simulink model "AC_Voltage_Controller_Bidirectional_L_Load"  (R2021b)
settings: Solver=ode23tb  StartTime=0.0  StopTime=0.1  MaxStep=1e-4  RelTol=1e-3
undefined symbols (not defined in the file): k, m
libraries: spsRMSLib x4, spsThyristorLib x4, spsVoltageMeasurementLib x4, spsACVoltageSourceLib x2, spsCurrentMeasurementLib x2, spsSeriesRLCBranchLib x2, spspowerguiLib x1
settings Model: Creator=90542  LastModifiedBy=90542

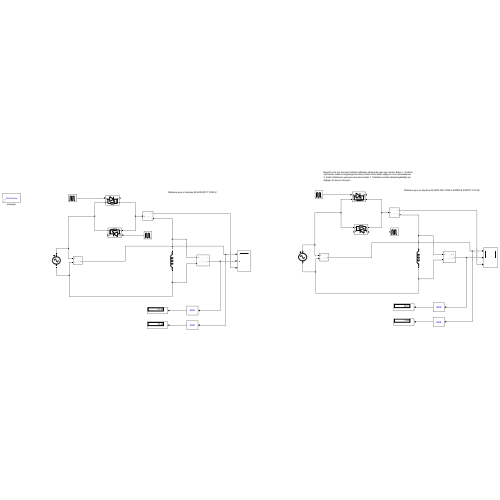
[thumbnail: Simulink's stored preview of the top-level diagram]
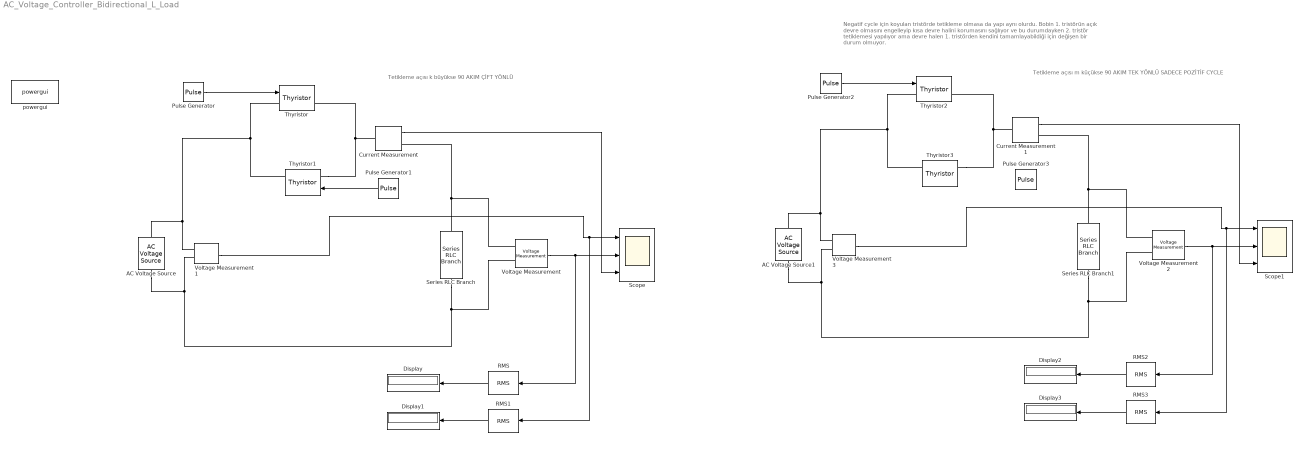
== system AC_Voltage_Controller_Bidirectional_L_Load ==
  note: Negatif cycle için koyulan tristörde tetikleme olmasa da yapı aynı olurdu. Bobin 1. tristörün açık devre olmasını engelleyip kısa devre halini korumasını sağlıyor ve bu durumdayken 2. tristör tetiklemesi yapılıyor ama devre halen 1. tristörden kendini tamamlayabildiği için değişen bir durum olmuyor.
  note: Tetikleme açısı m küçükse 90 AKIM TEK YÖNLÜ SADECE POZİTİF CYCLE
  note: Tetikleme açısı k büyükse 90 AKIM ÇİFT YÖNLÜ
  AC Voltage Source : spsACVoltageSourceLib/AC Voltage Source  Amplitude=100  Phase=0  Frequency=50  SampleTime=0  Measurements=None  BusType=swing  Pref=10e3  Qref=0  Qmin=-inf  Qmax=+inf
  AC Voltage Source1 : spsACVoltageSourceLib/AC Voltage Source  Amplitude=100  Phase=0  Frequency=50  SampleTime=0  Measurements=None  BusType=swing  Pref=10e3  Qref=0  Qmin=-inf  Qmax=+inf
  Current Measurement : spsCurrentMeasurementLib/Current Measurement  PhasorSimulation=off  OutputType=Complex  PSBequivalent=0
  Current Measurement1 : spsCurrentMeasurementLib/Current Measurement  PhasorSimulation=off  OutputType=Complex  PSBequivalent=0
  Display{,1..3} (4 alike) : Display
  Pulse Generator : DiscretePulseGenerator  PulseType=Time based  Amplitude=5  Period=0.02  PulseWidth=5  PhaseDelay=k*(0.02/360)
  Pulse Generator1 : DiscretePulseGenerator  PulseType=Time based  Amplitude=5  Period=0.02  PulseWidth=5  PhaseDelay=(k+180)*(0.02/360)
  Pulse Generator2 : DiscretePulseGenerator  PulseType=Time based  Amplitude=5  Period=0.02  PulseWidth=5  PhaseDelay=m*(0.02/360)
  Pulse Generator3 : DiscretePulseGenerator  PulseType=Time based  Amplitude=5  Period=0.02  PulseWidth=5  PhaseDelay=(m+180)*(0.02/360)
  RMS{,1..3} (4 alike) : spsRMSLib/RMS  TrueRMS=on  Freq=60  RMSInit=120  Ts=0
  Scope : Scope  NumInputPorts=3
  Scope1 : Scope  NumInputPorts=3
  Series RLC Branch : spsSeriesRLCBranchLib/Series RLC Branch  LConnTagsString=__new0  RConnTagsString=__new0  BranchType=L  Resistance=10  Inductance=10e-3  SetiL0=off  InitialCurrent=0  Capacitance=1e-6  Setx0=off  InitialVoltage=0  Measurements=None
  Series RLC Branch1 : spsSeriesRLCBranchLib/Series RLC Branch  LConnTagsString=__new0  RConnTagsString=__new0  BranchType=L  Resistance=10  Inductance=10e-3  SetiL0=off  InitialCurrent=0  Capacitance=1e-6  Setx0=off  InitialVoltage=0  Measurements=None
  Thyristor{,1..3} (4 alike) : spsThyristorLib/Thyristor  Ron=0.001  Lon=0  Vf=0.8  IC=0  Rs=500  Cs=250e-9  Measurements=on
  Voltage Measurement{,1..3} (4 alike) : spsVoltageMeasurementLib/Voltage Measurement  PhasorSimulation=off  OutputType=Complex  PSBequivalent=0
  powergui : spspowerguiLib/powergui  Priority=1  SimulationMode=Continuous  SampleTime=50e-6  frequency=60  Iterations=50  frequencyindice=50  Pbase=100e6  ErrMax=1e-4  UnitsV=kV  UnitsW=MW  buscounter=0  FunctionMessages=off  echomessages=off  EnableUseOfTLC=off  CurrentSourceSwitches=off  DisableSnubberDevices=off  DisableRonSwitches=off  DisableVfSwitches=off  DisplayEquations=off  AutomaticDiscreteSolvers=off  SolverType=Tustin/Backward Euler (TBE)  Interpol=off  ExternalGateDelay=off  methode=off  Ts=100  x0status=blocks  SPID=on  SwTol=0  HookPort=off  NonlinearTolerance=1e-4  nMaxIteration=100  ContinueOnMaxIteration=off  RestoreLinks=warning  ResistiveCurrentMeasurement=off  Frange=[0:2:500]  Ylog=off  Xlog=on  ShowGrid=off  save=off  variable=ZData  structure=0  ZoomFFT=off  StartTime=0.0  cycles=1  DisplayStyle=1  fundamental=60  FreqAxis=off  MaxFrequency=1000  frequencyindicesteady=1  RmsSteady=1  display=off
  wires:
  Pulse Generator/1 -> Thyristor/1
  Voltage Measurement/1 -> RMS/1, Scope/2
  Voltage Measurement1/1 -> RMS1/1, Scope/1
  Current Measurement/1 -> Scope/3
  RMS/1 -> Display/1
  Pulse Generator1/1 -> Thyristor1/1
  RMS1/1 -> Display1/1
  RMS2/1 -> Display2/1
  RMS3/1 -> Display3/1
  Voltage Measurement3/1 -> RMS3/1, Scope1/1
  Voltage Measurement2/1 -> RMS2/1, Scope1/2
  Current Measurement1/1 -> Scope1/3
  Pulse Generator2/1 -> Thyristor2/1
  connections:
  AC Voltage Source/RConn1 -- Thyristor1/RConn1 -- Thyristor/LConn1 -- Voltage Measurement1/LConn1
  AC Voltage Source/LConn1 -- Series RLC Branch/RConn1 -- Voltage Measurement/LConn2 -- Voltage Measurement1/LConn2
  Current Measurement/LConn1 -- Thyristor1/LConn1 -- Thyristor/RConn1
  Series RLC Branch/LConn1 -- Voltage Measurement/LConn1 -- Current Measurement/RConn1
  Series RLC Branch1/LConn1 -- Voltage Measurement2/LConn1 -- Current Measurement1/RConn1
  Current Measurement1/LConn1 -- Thyristor3/LConn1 -- Thyristor2/RConn1
  Voltage Measurement2/LConn2 -- Voltage Measurement3/LConn2 -- AC Voltage Source1/LConn1 -- Series RLC Branch1/RConn1
  AC Voltage Source1/RConn1 -- Thyristor3/RConn1 -- Thyristor2/LConn1 -- Voltage Measurement3/LConn1
